simulink model "engine_rpm"  (R2022b)
settings: Solver=ode45  StartTime=0.0  StopTime=50.0  FixedStep=0.001  RelTol=1e-3
PreLoadFcn:
  | load engine_rpm.mat
  | Iei = 0.022;
values from neighbouring files (symbols this model uses):
  ENGINE_SPEED = [800 1200 1600 2000 2400 2800 3200 3600 4000 4400 4800]    [engine_rpm.mat]    (also in ex3.mat)
  ENGINE_TORQUE = [-40 215 245 264 264 267 267 267 267 267 -44 117 ... (110 elements, 10x11)]    [engine_rpm.mat]    (also in ex3.mat)
  THROTTLE = [0 20 30 40 50 60 70 80 90 100]    [engine_rpm.mat]    (also in ex3.mat)
libraries: SignalEditorBlockLib x1
settings Model: Creator=nicholas  LastModifiedBy=bensweet
settings SolverCC: AlgebraicLoopSolver=TrustRegion  MaxZcPerStep=1
settings DataIOCC: ExternalInput=[t, T_impeller]  LimitDataPoints=on  LoadExternalInput=on  SaveFormat=Array  ReturnWorkspaceOutputs=off  SignalLoggingName=sigsOut
settings OptimizationCC: BlockReduction=off  BooleanDataType=off  OptimizeBlockIOStorage=off  BufferReuse=off  GlobalBufferReuse=off  ExpressionFolding=off  ExpressionDepthLimit=2147483647  LocalBlockOutputs=off  InitFltsAndDblsToZero=on  LifeSpan=inf  OptimizeDataStoreBuffers=off  BusAssignmentInplaceUpdate=off
settings DebuggingCC: CheckExecutionContextPreStartOutputMsg=on  UnconnectedInputMsg=warning  UnconnectedOutputMsg=warning  UnconnectedLineMsg=warning  PregeneratedLibrarySubsystemCodeDiagnostic=none  SFMachineParentedDataDiag=warning
settings HardwareCC: ProdBitPerPointer=32  ProdBitPerSizeT=32  ProdBitPerPtrDiffT=32  ProdLargestAtomicFloat=None  ProdIntDivRoundTo=Undefined  ProdEndianess=Unspecified  ProdWordSize=32  ProdHWDeviceType=32-bit Generic  TargetUnknown=on
settings ModelReferenceCC: EnableRefExpFcnMdlSchedulingChecks=on  PropagateSignalLabelsOutOfModel=off
settings SFSimCC: SimUseLocalCustomCode=off
settings RTWCC: RTWUseLocalCustomCode=off  DLArmComputeVersion=19.05
settings CodeAppCC: StateflowObjectComments=on
settings GRTTargetCC: TargetFcnLib=ansi_tfl_tmw.mat  TargetLangStandard=C89/C90 (ANSI)  CombineOutputUpdateFcns=off  GRTInterface=on
settings ConfigComp: CovMetricSettings=dw  CovSaveCumulativeToWorkspaceVar=on  CovSaveSingleToWorkspaceVar=on  CovExternalEMLEnable=off  CovSFcnEnable=off

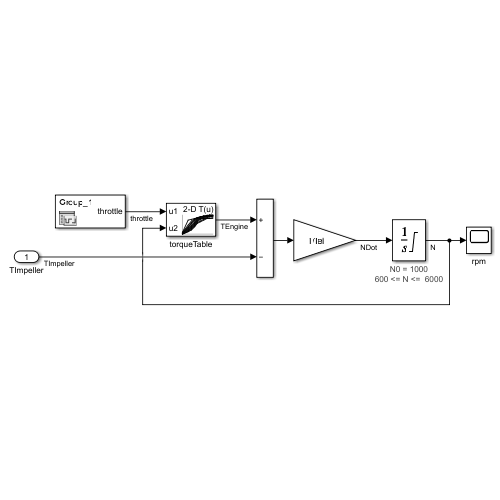
[thumbnail: Simulink's stored preview of the top-level diagram]
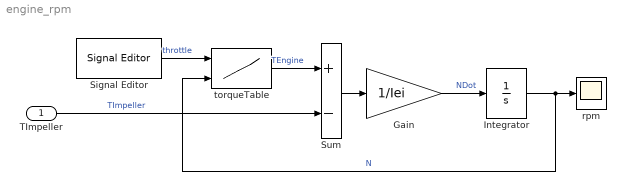
== system engine_rpm ==
  TImpeller : Inport
  Gain : Gain  Gain=1/Iei  SaturateOnIntegerOverflow=on  OutDataTypeStr=Inherit: Same as input  ParamDataTypeStr=Inherit: Same as input
  Integrator : Integrator  InitialCondition=1000  LimitOutput=on  UpperSaturationLimit=6000  LowerSaturationLimit=600
      settings: AttributesFormatString="N0 = %<InitialCondition>\\n%<LowerSaturationLimit> <= N <=  %<UpperSaturationLimit>\\n"
  Signal Editor : SignalEditorBlockLib/Signal Editor  FileName=engine_rpm_throttle_dataset.mat  ActiveScenario=Group_1  ActiveSignal=throttle  IsBus=off  OutputBusObjectStr=Bus: BusObject  SampleTime=0  ZeroCross=off  OutputAfterFinalValue=Extrapolation  Unit=inherit  PreserveSignalName=on
  Sum : Sum  Inputs=+-  InputSameDT=on  SaturateOnIntegerOverflow=on  OutDataTypeStr=Inherit: Same as first input
  rpm : Scope
  torqueTable : Lookup_n-D  BreakpointsForDimension1=THROTTLE  BreakpointsForDimension2=ENGINE_SPEED  Table=ENGINE_TORQUE  RndMeth=Simplest
      settings: InputPortMap=u0,u1
  wires:
  Sum/1 -> Gain/1
  Integrator/1 -> rpm/1, torqueTable/2  "N"
  Gain/1 -> Integrator/1  "NDot"
  TImpeller/1 -> Sum/2  "TImpeller"
  torqueTable/1 -> Sum/1  "TEngine"
  Signal Editor/1 -> torqueTable/1  "throttle"
